simulink model "parametrized_lunar_landing_modified"  (R2016b)
settings: Solver=ode5  StartTime=0.0  StopTime=100  FixedStep=0.01  RelTol=1e-3
settings Model: Creator=Thomas  LastModifiedBy=Thomas
settings DataIOCC: SaveFormat=StructureWithTime  SaveOutput=off  SaveTime=off

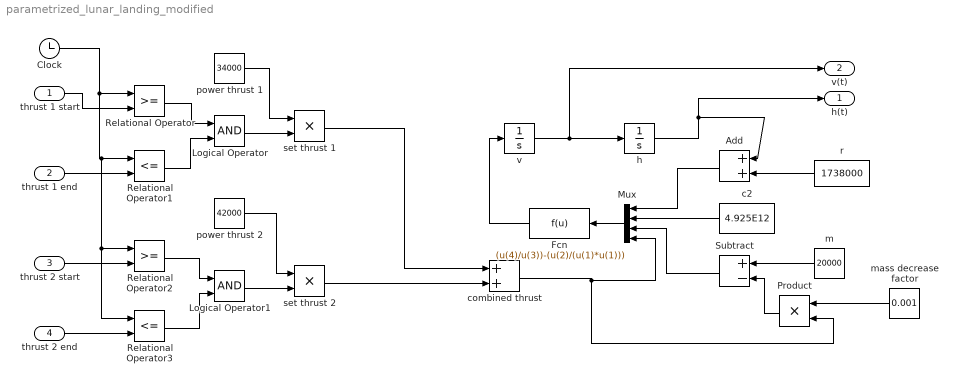
== system parametrized_lunar_landing_modified ==
  thrust 1 start : Inport
  thrust 1 end : Inport  Port=2
  thrust 2 start : Inport  Port=3
  thrust 2 end : Inport  Port=4
  Add : Sum
  Clock : Clock
  Fcn : Fcn  Expr=(u(4)/u(3))-(u(2)/(u(1)*u(1)))
  Logical Operator : Logic  AllPortsSameDT=off  OutDataTypeStr=boolean
  Logical Operator1 : Logic  AllPortsSameDT=off  OutDataTypeStr=boolean
  Mux : Mux
  Product : Product
  Relational Operator : RelationalOperator  OutDataTypeStr=boolean  RndMeth=Simplest
  Relational Operator1 : RelationalOperator  Operator=<=  OutDataTypeStr=boolean  RndMeth=Simplest
  Relational Operator2 : RelationalOperator  OutDataTypeStr=boolean  RndMeth=Simplest
  Relational Operator3 : RelationalOperator  Operator=<=  OutDataTypeStr=boolean  RndMeth=Simplest
  Subtract : Sum  Inputs=+-
  c2 : Constant  Value=4.925E12
  combined thrust : Sum
  h : Integrator  InitialCondition=1000
  m : Constant  Value=20000
  mass decrease factor : Constant  Value=0.001
  power thrust 1 : Constant  Value=34000
  power thrust 2 : Constant  Value=42000
  r : Constant  Value=1738000
  set thrust 1 : Product
  set thrust 2 : Product
  v : Integrator  InitialCondition=-10
  h(t) : Outport
  v(t) : Outport  Port=2
  wires:
  v/1 -> h/1, v(t)/1
  Mux/1 -> Fcn/1
  h/1 -> h(t)/1, Add/1
  r/1 -> Add/2
  Add/1 -> Mux/1
  c2/1 -> Mux/2
  combined thrust/1 -> Mux/4, Product/2
  Fcn/1 -> v/1
  Clock/1 -> Relational Operator3/1, Relational Operator2/1, Relational Operator1/1, Relational Operator/1
  thrust 1 start/1 -> Relational Operator/2
  thrust 1 end/1 -> Relational Operator1/2
  Relational Operator/1 -> Logical Operator/1
  Relational Operator1/1 -> Logical Operator/2
  power thrust 1/1 -> set thrust 1/1
  Logical Operator/1 -> set thrust 1/2
  thrust 2 start/1 -> Relational Operator2/2
  thrust 2 end/1 -> Relational Operator3/2
  Relational Operator2/1 -> Logical Operator1/1
  Relational Operator3/1 -> Logical Operator1/2
  Logical Operator1/1 -> set thrust 2/2
  set thrust 1/1 -> combined thrust/1
  set thrust 2/1 -> combined thrust/2
  power thrust 2/1 -> set thrust 2/1
  mass decrease factor/1 -> Product/1
  m/1 -> Subtract/1
  Product/1 -> Subtract/2
  Subtract/1 -> Mux/3
